simulink model "full_boat_system"  (R2025b)
settings: Solver=FixedStepAuto  StartTime=0.0  StopTime=90  RelTol=1e-3  EnableMultiTasking=on
libraries: arduinolib x9, arduinowifilib x4, dspnetwork x3
settings Model: ExtModeTrigDuration=2  Creator=M  LastModifiedBy=M
settings SolverCC: AutoInsertRateTranBlk=on
settings OptimizationCC: EnhancedBackFolding=on  PassReuseOutputArgsAs=Individual arguments  ZeroExternalMemoryAtStartup=off  ZeroInternalMemoryAtStartup=off  MaxStackSize=64  OptimizeBlockOrder=speed  DifferentSizesBufferReuse=on  OptimizationCustomize=off  EfficientTunableParamExpr=on
settings DebuggingCC: ParameterTunabilityLossMsg=error
settings HardwareCC: ProdBitPerInt=16.0  ProdBitPerPointer=16.0  ProdBitPerSizeT=16.0  ProdBitPerPtrDiffT=16.0  ProdLargestAtomicFloat=None  ProdWordSize=8.0  ProdHWDeviceType=Atmel->AVR  UseEmbeddedCoderFeatures=off  UseSimulinkCoderFeatures=off
settings SFSimCC: MATLABDynamicMemAlloc=off
settings RTWCC: SystemTargetFile=ert.tlc  HardwareBoard=Arduino Uno  TLCOptions="-aInlineSetEventsForThisBaseRateFcn=TLC_FALSE -aSuppressMultiTaskScheduler=TLC_FALSE   -aRateBasedStepFcn=1"  TemplateMakefile=ert_default_tmf  Toolchain=Arduino AVR  BuildConfiguration=Faster Runs  Description=Embedded Coder
settings CodeAppCC: ForceParamTrailComments=on  IgnoreCustomStorageClasses=off  OperatorAnnotations=on  SimulinkDataObjDesc=on  SFDataObjDesc=on  InsertBlockDesc=on
settings ERTTargetCC: ExtModeTransport=3.0  ExtModeStaticAlloc=on  ExtModeAutomaticAllocSize=off  ExtModeStaticAllocSize=250.0  ExtModeMexFile=ext_xcp  ExtModeIntrfLevel=Level2 - Open  InlinedParameterPlacement=Hierarchical  SupportContinuousTime=on  SupportNonInlinedSFcns=on  SupportVariableSizeSignals=on

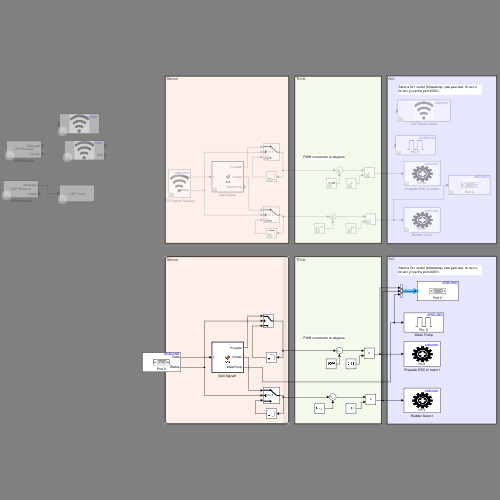
[thumbnail: Simulink's stored preview of the top-level diagram]
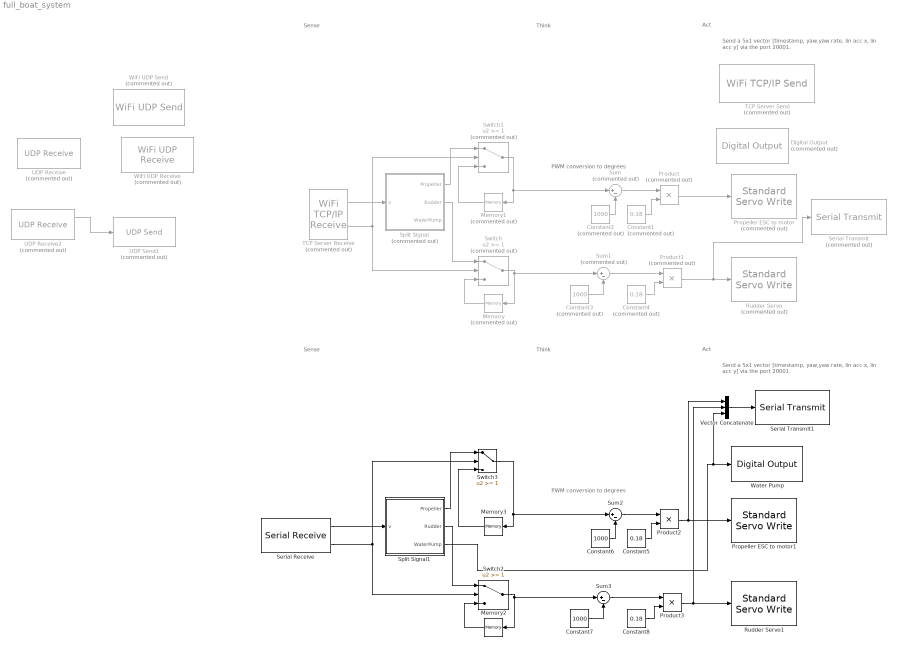
== system full_boat_system ==
  note: Think
  note: PWM conversion to degrees
  note: Send a 5x1 vector [timestamp, yaw,yaw rate, lin acc x, lin acc y] via the port 20001.
  note: Sense
  note: Act
  note: PWM conversion to degrees
  note: Sense
  note: Send a 5x1 vector [timestamp, yaw,yaw rate, lin acc x, lin acc y] via the port 20001.
  note: Think
  note: Act
  Constant1 : Constant  Commented=on  Value=0.18  OutDataTypeStr=single
  Constant2 : Constant  Commented=on  Value=1000  OutDataTypeStr=single
  Constant3 : Constant  Commented=on  Value=1000  OutDataTypeStr=single
  Constant4 : Constant  Commented=on  Value=0.18  OutDataTypeStr=single
  Constant5 : Constant  Value=0.18  OutDataTypeStr=single
  Constant6 : Constant  Value=1000  OutDataTypeStr=single
  Constant7 : Constant  Value=1000  OutDataTypeStr=single
  Constant8 : Constant  Value=0.18  OutDataTypeStr=single
  Digital Output : arduinolib/Digital Output  Commented=on  pinNumber=9  Direction=output  blockPlatform=arduino
      settings: LibrarySourceBlock=gizmoLibrary/Arduino Utilities/Digital Output
  Memory : Memory  Commented=on  InitialCondition=1500
  Memory1 : Memory  Commented=on  InitialCondition=1500
  Memory2 : Memory  InitialCondition=1500
  Memory3 : Memory  InitialCondition=1500
  Product : Product  Commented=on  OutDataTypeStr=single  RndMeth=Nearest
  Product1 : Product  Commented=on  OutDataTypeStr=single  RndMeth=Nearest
  Product2 : Product  OutDataTypeStr=single  RndMeth=Nearest
  Product3 : Product  OutDataTypeStr=single  RndMeth=Nearest
  Propeller ESC to motor : arduinolib/Standard Servo Write  Commented=on  pinNumber=26  ServoIndex=0  blockPlatform=ESP32
  Propeller ESC to motor1 : arduinolib/Standard Servo Write  pinNumber=6  ServoIndex=0  blockPlatform=ESP32
  Rudder Servo : arduinolib/Standard Servo Write  Commented=on  pinNumber=25  ServoIndex=1  blockPlatform=ESP32
  Rudder Servo1 : arduinolib/Standard Servo Write  pinNumber=3  ServoIndex=1  blockPlatform=ESP32
  Serial Receive : arduinolib/Serial Receive  portNumber=0  DataType=single  blockPlatform=ARDUINO  TimeOut=0  MaxDataLength=10  isARMArch=off  DataLengthOption=Length via dialog  Datalength=12  Header=[]  Terminator=[]  SampleTime=0.2  ShowOutStatus=on
  Serial Transmit : arduinolib/Serial Transmit  Commented=on  portNumber=0  sendmode=println  label=prop=  sendformat=Decimal  floatprecision=1  header=[]  terminator=[]  blockPlatform=ARDUINO
  Serial Transmit1 : arduinolib/Serial Transmit  portNumber=0  sendmode=println  label=msg =  sendformat=Decimal  floatprecision=1  header=[]  terminator=[]  blockPlatform=ARDUINO
  Split Signal : MATLAB Function  Commented=on  TreatAsAtomicUnit=on
  Split Signal1 : MATLAB Function  TreatAsAtomicUnit=on
  Sum : Sum  Commented=on  Inputs=|+-  OutDataTypeStr=single  RndMeth=Nearest
  Sum1 : Sum  Commented=on  Inputs=|+-  OutDataTypeStr=single  RndMeth=Nearest
  Sum2 : Sum  Inputs=|+-  OutDataTypeStr=single  RndMeth=Nearest
  Sum3 : Sum  Inputs=|+-  OutDataTypeStr=single  RndMeth=Nearest
  Switch : Switch  Commented=on  Threshold=1  RndMeth=Nearest  SaturateOnIntegerOverflow=off  InputSameDT=off
  Switch1 : Switch  Commented=on  Threshold=1  RndMeth=Nearest  SaturateOnIntegerOverflow=off  InputSameDT=off
  Switch2 : Switch  Threshold=1  RndMeth=Nearest  SaturateOnIntegerOverflow=off  InputSameDT=off
  Switch3 : Switch  Threshold=1  RndMeth=Nearest  SaturateOnIntegerOverflow=off  InputSameDT=off
  TCP Server Receive : arduinowifilib/WiFi TCP//IP Receive  Commented=on  Mode_=Server  serverport=20001  RemoteAddr_=192.168.137.1  RemoteServerPort_=10000  DataType_=single  DataSize_=2  SampleTime_=0.02  remoteipoctet1=192  remoteipoctet2=168  remoteipoctet3=137  remoteipoctet4=1  wifiTCPServerIndex=0  wifiTCPClientIndex=0  blockPlatform=ARDUINO  isARMArch=false  BlockingMode_=off  BlockTimeout_=0.03
  TCP Server Send : arduinowifilib/WiFi TCP//IP Send  Commented=on  Mode_=Server  serverport=20001  RemoteAddr_=192.168.137.1  RemoteServerPort_=10000  remoteipoctet1=192  remoteipoctet2=168  remoteipoctet3=137  remoteipoctet4=1  wifiTCPServerIndex=0  wifiTCPClientIndex=0  blockPlatform=ARDUINO  isARMArch=false
  UDP Receive : dspnetwork/UDP Receive  Commented=on  localURL='0.0.0.0'  localPort=20000  remoteURL='192.168.137.1'  remotePort=-1  recvBufferSize=32  dims=32  signalDatatype=single  isComplex=off  isVarSize=off  showBlockingTime=off  blockingTime=0  sampletime=0.02  blockPlatform=[]
      settings: LibrarySourceBlock=dspsrcs4/UDP Receive
  UDP Receive2 : dspnetwork/UDP Receive  Commented=on  localURL='0.0.0.0'  localPort=20000  remoteURL='192.168.137.1'  remotePort=-1  recvBufferSize=8192  dims=255  signalDatatype=uint8  isComplex=off  isVarSize=off  showBlockingTime=off  blockingTime=0  sampletime=0.02  blockPlatform=[]
      settings: LibrarySourceBlock=dspsrcs4/UDP Receive
  UDP Send1 : dspnetwork/UDP Send  Commented=on  remoteURL='192.168.137.1'  remotePort=10000  localURL='0.0.0.0'  localPortSource=Specify via dialog  localPort=20000  sendBufferSize=8192  sampletime=-1  blockPlatform=[]  separateLengthPort=0
      settings: LibrarySourceBlock=dspsnks4/UDP Send
  Vector Concatenate : Concatenate  NumInputs=3
  Water Pump : arduinolib/Digital Output  pinNumber=9  Direction=output  blockPlatform=arduino
      settings: LibrarySourceBlock=gizmoLibrary/Arduino Utilities/Digital Output
  WiFi UDP Receive : arduinowifilib/WiFi UDP Receive  Commented=on  localport=20000  DataType=single  DataLength=1  SampleTime_=-1  wifiUDPIndex=0  blockPlatform=ARDUINO  isARMArch=false
  WiFi UDP Send : arduinowifilib/WiFi UDP Send  Commented=on  remoteIPOctetString=192.168.137.1  remoteport=10000  localport=20000  remoteipoctet1=192  remoteipoctet2=168  remoteipoctet3=137  remoteipoctet4=1  wifiUDPIndex=0  blockPlatform=ARDUINO  isARMArch=false
  wires:
  Sum1/1 -> Product1/1
  UDP Receive2/1 -> UDP Send1/1
  Constant2/1 -> Sum/2
  Sum/1 -> Product/1
  Constant1/1 -> Product/2
  Constant4/1 -> Product1/2
  TCP Server Receive/2 -> Switch1/2, Switch/2
  Split Signal/2(Rudder) -> Switch/1
  Switch/1 -> Sum1/1, Memory/1
  Memory/1 -> Switch/3
  Memory1/1 -> Switch1/3
  Constant3/1 -> Sum1/2
  Switch1/1 -> Sum/1, Memory1/1
  TCP Server Receive/1 -> Split Signal/1(v)
  Split Signal/1(Propeller) -> Switch1/1
  Product/1 -> Propeller ESC to motor/1
  Product1/1 -> Serial Transmit/1, Rudder Servo/1
  Split Signal1/1(Propeller) -> Switch3/1
  Memory3/1 -> Switch3/3
  Product3/1 -> Vector Concatenate/2, Rudder Servo1/1
  Serial Receive/2 -> Switch2/2, Switch3/2
  Constant6/1 -> Sum2/2
  Sum3/1 -> Product3/1
  Constant8/1 -> Product3/2
  Switch3/1 -> Sum2/1, Memory3/1
  Serial Receive/1 -> Split Signal1/1(v)
  Sum2/1 -> Product2/1
  Switch2/1 -> Sum3/1, Memory2/1
  Memory2/1 -> Switch2/3
  Constant7/1 -> Sum3/2
  Product2/1 -> Vector Concatenate/1, Propeller ESC to motor1/1
  Constant5/1 -> Product2/2
  Split Signal1/2(Rudder) -> Switch2/1
  Split Signal1/3(WaterPump) -> Vector Concatenate/3, Water Pump/1
  Vector Concatenate/1 -> Serial Transmit1/1

== matlab function full_boat_system/Split Signal ==
  data: v input; Propeller output; Rudder output; WaterPump output
function [Propeller,Rudder,WaterPump] = fcn(v)

Propeller = v(1);
Rudder = v(2);
WaterPump = v(3);

end

== matlab function full_boat_system/Split Signal1 ==
  data: v input; Propeller output; Rudder output; WaterPump output
function [Propeller,Rudder,WaterPump] = fcn(v)

Propeller = v(1);
Rudder = v(2);
WaterPump = v(3);

end
